simulink model "slexClassificationECOCPredictExample"  (R2023a)
settings: Solver=FixedStepDiscrete  StartTime=0.0  StopTime=activityInput.time(end)  FixedStep=1  RelTol=1e-3
PreLoadFcn:
  | if ~exist("ecocMdl","var")
  | 
  | load humanactivity
  | X = feat;
  | Y = actid;
  | 
  | rng("default") % For reproducibility of the partition
  | cv = cvpartition(Y,"Holdout",0.20);
  | trainingInds = training(cv);
  | testInds = test(cv);
  | XTrain = X(trainingInds,:);
  | YTrain = Y(trainingInds);
  | XTest = X(testInds,:);
  | YTest = Y(testInds);
  | 
  | ecocMdl = fitcecoc(XTrain,YTrain);
  | 
  | [nTest,p] = size(XTest);
  | activityInput.time = (0:(nTest-1))';
  | activityInput.signals(1).values = XTest;
  | activityInput.signals(1).dimensions = p;
  | 
  | end
libraries: statsLibrary x1
settings Model: Creator=The MathWorks, Inc.  LastModifiedBy=The MathWorks, Inc.
settings DataIOCC: ExternalInput=activityInput  LoadExternalInput=on
settings OptimizationCC: ReuseModelBlockBuffer=off

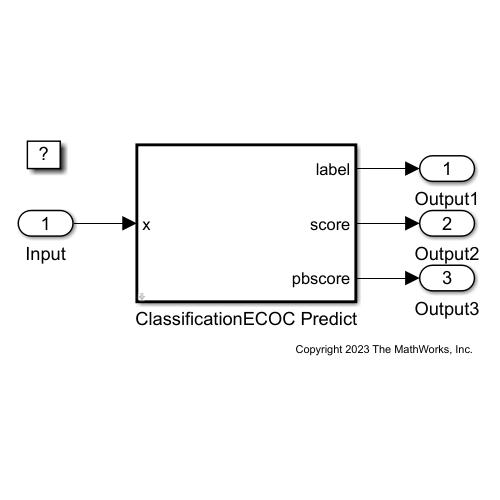
[thumbnail: Simulink's stored preview of the top-level diagram]
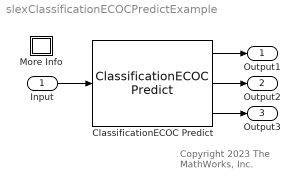
== system slexClassificationECOCPredictExample ==
  note: Copyright 2023 The MathWorks, Inc.
  Input : Inport
  ClassificationECOC Predict : statsLibrary/Classification/ClassificationECOC Predict  TrainedLearner=ecocMdl  ShowOutputScore=on  ShowOutputPBScore=on  BinaryLoss=hinge  Decoding=lossweighted  LabelDataTypeStr=Inherit: Inherit via back propagation  LabelOutMin=[]  LabelOutMax=[]  ScoreOutMin=[]  ScoreOutMax=[]  PBScoreOutMin=[]  PBScoreOutMax=[]  KernelDataTypeStr=double  KernelOutMin=[]  KernelOutMax=[]  InnerProductOutMin=[]  InnerProductOutMax=[]  StoredEnumName=ecocMdl_enumLabels
  More Info : Subsystem
      settings: OpenFcn=showExample('stats/PredictClassLabelsUsingClassificationECOCPredictBlockExample')
      mask Display: disp('?')
  Output1 : Outport
  Output2 : Outport  Port=2
  Output3 : Outport  Port=3
  wires:
  ClassificationECOC Predict/1 -> Output1/1
  ClassificationECOC Predict/2 -> Output2/1
  ClassificationECOC Predict/3 -> Output3/1
  Input/1 -> ClassificationECOC Predict/1

== system slexClassificationECOCPredictExample/More Info ==
